simulink model "lookupTableDynamic_TestGen40"  (R2017b)
settings: Solver=FixedStepDiscrete  StartTime=0.0  StopTime=10.0  RelTol=1e-3
libraries: simulink x1
settings Model: Creator=ktrinh  LastModifiedBy=ktrinh
settings DebuggingCC: ParameterOverflowMsg=none

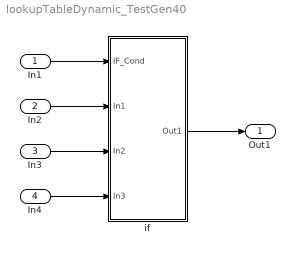
== system lookupTableDynamic_TestGen40 ==
  In1 : Inport
  In2 : Inport  Port=2
  In3 : Inport  Port=3
  In4 : Inport  Port=4
  if : Subsystem  AncestorBlock=Block_TestLib/if
  Out1 : Outport
  wires:
  In1/1 -> if/1(IF_Cond)
  In2/1 -> if/2(In1)
  In3/1 -> if/3(In2)
  In4/1 -> if/4(In3)
  if/1(Out1) -> Out1/1

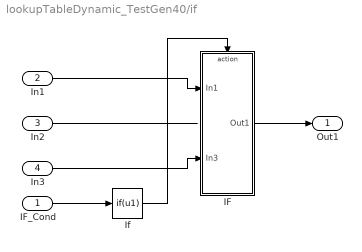
== system lookupTableDynamic_TestGen40/if ==
  IF_Cond : Inport  OutDataTypeStr=boolean
  In1 : Inport  Port=2
  In2 : Inport  Port=3
  In3 : Inport  Port=4
  IF : Subsystem  TreatAsAtomicUnit=on
  If : If  IfExpression=u1  ShowElse=off
  Out1 : Outport
  wires:
  If/1 -> IF/Action
  In1/1 -> IF/1(In1)
  In2/1 -> ?
  In3/1 -> IF/2(In3)
  IF_Cond/1 -> If/1
  IF/1(Out1) -> Out1/1

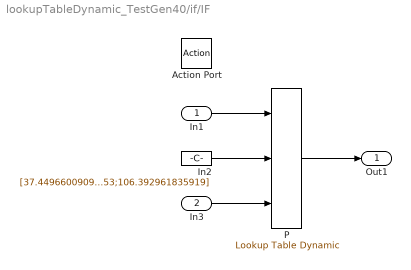
== system lookupTableDynamic_TestGen40/if/IF ==
  In1 : Inport  OutMin=35.4497  OutMax=108  OutDataTypeStr=uint32  PortDimensions=1
  In3 : Inport  Port=2  PortDimensions=5
  Action Port : ActionPort  ActionType=then
  In2 : Constant  Value=[37.4496600909735;44.1610364040487;58.0224243619452;77.7110808912453;106.392961835919]  OutDataTypeStr=uint32
  P : simulink/Lookup Tables/Lookup Table Dynamic  LookUpMeth=Use Input Above  OutDataType=fixdt('uint8')  OutScaling=[]  OutputDataTypeScalingMode=Specify via dialog  OutDataTypeStr=uint8  RndMeth=Simplest  DoSatur=off
      settings: SourceProductName=Simulink
  Out1 : Outport
  wires:
  In1/1 -> P/1
  In2/1 -> P/2
  In3/1 -> P/3
  P/1 -> Out1/1
